simulink model "Unicycle_model"  (R2020b)
settings: Solver=VariableStepAuto  StartTime=0.0  StopTime=20.0  RelTol=1e-3
InitFcn:
  | if ~exist('x0')
  |   x0 = [0 0 0];
  |   msgbox(sprintf('x0 not defined in workspace, setting it to [%g %g %g]\n', x0));
  | end
  | if ~exist('L')
  |   L = [1 -1 0];
  |   msgbox(sprintf('L not defined in workspace, setting it to [%g %g %g]\n', L));
  | end
  | % clean up old vehicle icons
  | set(0, 'ShowHiddenHandles', 'on')
  | delete(findobj('Tag', 'vehicle'))
  | set(0, 'ShowHiddenHandles', 'off')
StopFcn:
  | % update the XY scope
  | set(0, 'ShowHiddenHandles', 'on')
  | fig = findobj('name', 'XY');
  | ax = findobj(fig, 'type', 'axes');
  | axes(ax)
  | grid on
  | hold on
  | %plot_vehicle(x0, 'g', 'Tag', 'vehicle')
  | %plot_homline(L, 'r--', 'Tag', 'vehicle')
  | hold off
  | set(0, 'ShowHiddenHandles', 'off')
settings Model: Creator=nandi  LastModifiedBy=nandi

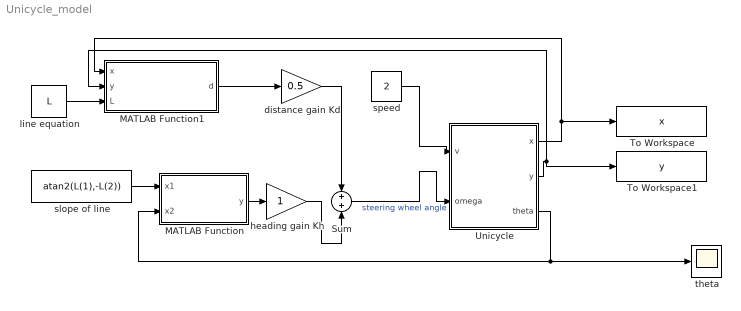
== system Unicycle_model ==
  MATLAB Function : MATLAB Function  TreatAsAtomicUnit=on
  MATLAB Function1 : MATLAB Function  TreatAsAtomicUnit=on
  Sum : Sum
  To Workspace : ToWorkspace  VariableName=x  SampleTime=-1
      settings: Save2DSignal=2-D array (concatenate along first dimension)
  To Workspace1 : ToWorkspace  VariableName=y  SampleTime=-1
      settings: Save2DSignal=2-D array (concatenate along first dimension)
  Unicycle : Subsystem  mask{vl=1, al=1, x0=x0, ol=Inf}
      mask prompts: vl "V_limit"; al "A_limit"; x0 "Initial state (x,y,theta)"; ol "omega_limit"
      mask Display:
      | port_label('input', 1, 'v')
      | port_label('input', 2, 'omega')
      | port_label('output', 1, 'x')
      | port_label('output', 2, 'y')
      | port_label('output', 3, 'theta')
  distance gain Kd : Gain  Gain=0.5
  heading gain Kh : Gain
  line equation : Constant  Value=L
  slope of line : Constant  Value=atan2(L(1),-L(2))
  speed : Constant  Value=2  VectorParams1D=off  SampleTime=0.02
  theta : Scope
  wires:
  Unicycle/3(theta) -> MATLAB Function/2(x2), theta/1
  Unicycle/1(x) -> To Workspace/1, MATLAB Function1/1(x)
  distance gain Kd/1 -> Sum/1
  line equation/1 -> MATLAB Function1/3(L)
  Unicycle/2(y) -> To Workspace1/1, MATLAB Function1/2(y)
  Sum/1 -> Unicycle/2(omega)  "steering wheel angle"
  heading gain Kh/1 -> Sum/2
  speed/1 -> Unicycle/1(v)
  MATLAB Function/1(y) -> heading gain Kh/1
  slope of line/1 -> MATLAB Function/1(x1)
  MATLAB Function1/1(d) -> distance gain Kd/1

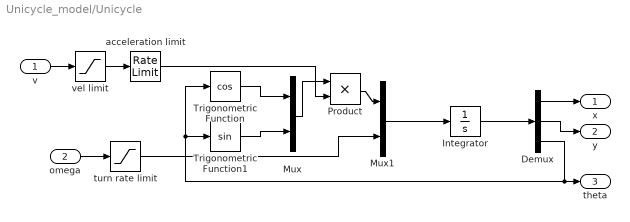
== system Unicycle_model/Unicycle ==
  v : Inport
  omega : Inport  Port=2
  Demux : Demux  Outputs=3
  Integrator : Integrator  InitialCondition=x0
  Mux : Mux  Inputs=2
  Mux1 : Mux  Inputs=2
  Product : Product  RndMeth=Zero
  Trigonometric Function : Trigonometry  Operator=cos
  Trigonometric Function1 : Trigonometry
  acceleration limit : RateLimiter  RisingSlewLimit=al  FallingSlewLimit=-al  SampleTimeMode=inherited
  turn rate limit : Saturate  UpperLimit=ol  LowerLimit=-ol
  vel limit : Saturate  UpperLimit=vl  LowerLimit=-vl
  x : Outport  VectorParamsAs1DForOutWhenUnconnected=off
  y : Outport  Port=2  VectorParamsAs1DForOutWhenUnconnected=off
  theta : Outport  Port=3  VectorParamsAs1DForOutWhenUnconnected=off
  wires:
  Demux/3 -> theta/1, Trigonometric Function1/1, Trigonometric Function/1
  Demux/2 -> y/1
  Demux/1 -> x/1
  Trigonometric Function/1 -> Mux/1
  vel limit/1 -> acceleration limit/1
  Product/1 -> Mux1/1
  v/1 -> vel limit/1
  omega/1 -> turn rate limit/1
  acceleration limit/1 -> Product/2
  Mux/1 -> Product/1
  Integrator/1 -> Demux/1
  turn rate limit/1 -> Mux1/2
  Mux1/1 -> Integrator/1
  Trigonometric Function1/1 -> Mux/2

== matlab function Unicycle_model/MATLAB Function ==
  data: x1 input; y output; x2 input
function y = ang_diff(x1,x2)

y = angdiff(x1,x2);

== matlab function Unicycle_model/MATLAB Function1 ==
  data: x input; y input; d output; L input
function d = dist_from_line(x,y,L)
d = (x*L(1)+y*L(2)+L(3))/sqrt(L(1)^2+L(2)^2);
